simulink model "Ford_T3T6_ArchCnctnDigrm"  (R2016b)
settings: Solver=FixedStepDiscrete  StartTime=0.0  StopTime=10.0  RelTol=1e-3  EnableMultiTasking=on
libraries: canmsglib x15
(part 7 of 15)

== system Ford_T3T6_ArchCnctnDigrm/Vector Components Base Software/SYS ==
  AR001ABswM_BswM : Subsystem  Tag=0.0.X  Description=The BSW Mode Manager is the module that implements the part of the Vehicle Mode Management and Application Mode Management concept that resides in the BSW. Its responsibility is to arbitrate mode requests from application layer SW-Cs or other BSW modules based on simple rules, and perform actions based on the arbitration result.
      settings: AttributesFormatString=Version: %<Tag>
  AR001AComM_ComM : Subsystem  Tag=0.0.X  Description=The Communication Manager Module (COM Manager, ComM) is a component of the Basic Software (BSW). It is a Resource Manager, which encapsulates the control of the underlying communication services. The ComM module controls basic software modules relating to communication and not software components or runnable entities. The ComM module collects the bus communication access requests from communication requestors and coordinates the bus communication access requests. The purpose of the ComM module is: 1. Simplifying the usage of the bus communication stack for the user. This includes a simplified network management handling. 2. Coordinating the availability of the bus communication stack (allow sending and receiving of signals) of multiple independent software components on one ECU. 3. Offer an API to disable sending of signals to prevent the ECU from (actively) waking up the communication bus. 4. Controlling of more than one communication bus channel of an ECU by implementing a channel state machine for every channel. 5. Offering the possibility to force an ECU that keeps the bus awake to the ï¿½No Communicationï¿½ mode. 6. Simplifying the resource management by allocating all resources necessary for the requested Communication Mode.
      settings: AttributesFormatString=Version: %<Tag>
  AR001ADet_Det : Subsystem  Tag=0.0.X  Description=All detected development errors in the Basic Software are reported to this module. The API parameters allow for tracing source and kind of error: Module in which error has been detected, Function in which error has been detected, Type of error
      settings: AttributesFormatString=Version: %<Tag>
  AR001AWdgIf_WdgIf : Subsystem  Tag=0.0.X  Description=In case of more than one watchdog device and watchdog driver (e.g. both an internal software watchdog and an external hardware watchdog) being used on an ECU, this module allows the watchdog manager (or any other client of the watchdog) to select the correct watchdog driver - and thus the watchdog device - while retaining the API and functionality of the underlying driver.
      settings: AttributesFormatString=Version: %<Tag>
  AR001AWdgM_WdgM : Subsystem  Tag=0.0.X  Description=The Watchdog Manager is able to supervise the program execution abstracting from the triggering of hardware watchdog entities. The Watchdog Manager supervises the execution of a configurable number of socalled Supervised Entities. When it detects a violation of the configured temporal and/or logical constraints on program execution, it takes a number of configurable actions to recover from this failure. The watchdog Manager provides three mechanisms: 1. Alive supervision ï¿½ for supervision of timing of periodic software. 2. Deadline monitoring ï¿½ for aperiodic software. 3. Logical monitoring ï¿½ for supervision of the correctness of the execution sequence.
      settings: AttributesFormatString=Version: %<Tag>
  tag scope: BswM_RequestMode=global, ComM_RequestComMode=global, PortDefinedArgument_CheckpointReached=global, WdgM_ActivateSupervisionEntity=global, WdgM_CheckpointReached=global, WdgM_DeactivateSupervisionEntity=global
  wires:
  AR001ABswM_BswM/1(BswM_RequestMode) -> [BswM_RequestMode]
  AR001AComM_ComM/1(ComM_RequestComMode) -> [ComM_RequestComMode]
  AR001AWdgM_WdgM/1(PortDefinedArgument_CheckpointReached) -> [PortDefinedArgument_CheckpointReached]
  AR001AWdgM_WdgM/2(WdgM_ActivateSupervisionEntity) -> [WdgM_ActivateSupervisionEntity]
  AR001AWdgM_WdgM/3(WdgM_CheckpointReached) -> [WdgM_CheckpointReached]
  AR001AWdgM_WdgM/4(WdgM_DeactivateSupervisionEntity) -> [WdgM_DeactivateSupervisionEntity]

== system Ford_T3T6_ArchCnctnDigrm/Vehicle Com/CF049A_FordVehSpdArbn ==
  FordAbsModlPrsnt : Inport
  FordEscModlPrsnt : Inport  Port=2
  FordVehFrntLeWhlSpd : Inport  Port=3
  FordVehFrntLeWhlSpdVld : Inport  Port=4
  FordVehFrntRiWhlSpd : Inport  Port=5
  FordVehFrntRiWhlSpdVld : Inport  Port=6
  FordVehReLeWhlSpd : Inport  Port=7
  FordVehReLeWhlSpdVld : Inport  Port=8
  FordVehReRiWhlSpd : Inport  Port=9
  FordVehReRiWhlSpdVld : Inport  Port=10
  FordVehSpdBrkModl : Inport  Port=11
  FordVehSpdBrkModlLoQlyVld : Inport  Port=12
  FordVehSpdBrkModlVld : Inport  Port=13
  FordVehSpdEngModl : Inport  Port=14
  FordVehSpdEngModlLoQlyVld : Inport  Port=15
  FordVehSpdEngModlVld : Inport  Port=16
  FordVehTireCircum_GetErrorStatus : Inport  Port=17
  FordVehSpd : Outport
  FordVehSpdLoQly : Outport  Port=2
  FordVehSpdLoQlyVld : Outport  Port=3
  FordVehSpdVld : Outport  Port=4

== system Ford_T3T6_ArchCnctnDigrm/Vehicle Com/CF100A_FordCanSigVldFlgGenr ==
  ActvFrntSteerModlSteerWhlAgVldInt : Inport
  FordVehActvFrntSteerModSteerWhlAgRaw : Inport  Port=2
  FordVehGearLvrPosnRaw : Inport  Port=3
  FordVehGearPosnRaw : Inport  Port=4
  FordVehParkAidModlReqdAgRaw : Inport  Port=5
  FordVehParkAidModlReqdStsRaw : Inport  Port=6
  FordVehTrlrAgOffsDirRaw : Inport  Port=7
  FordVehTrlrAidIdnNrRaw : Inport  Port=8
  FordVehTrlrAidSetUpRaw : Inport  Port=9
  FordVehTrlrAidTrlrRvsGuidcStsRaw : Inport  Port=10
  FordVehTrlrEnaReqRaw : Inport  Port=11
  FordVehTrlrIdnTypRaw : Inport  Port=12
  FordVehTrlrRvsCnclReqRaw : Inport  Port=13
  FordVehTrlrRvsEnaRaw : Inport  Port=14
  FordVehTrlrRvsMsgTxtReqRaw : Inport  Port=15
  FordVehTrsmDesGearRaw : Inport  Port=16
  GearLvrPosnVldInt : Inport  Port=17
  GearPosnRawVldInt : Inport  Port=18
  ImgProcgDataPrsntInt : Inport  Port=19
  ParkAidModlReqdAgVldInt : Inport  Port=20
  ParkAidModlReqdStsVldInt : Inport  Port=21
  TrlrAidDataPrsntInt : Inport  Port=22
  TrlrAidDataThreePrsntInt : Inport  Port=23
  TrlrAidStsThreePrsntInt : Inport  Port=24
  TrsmDesGearRawVldInt : Inport  Port=25
  FordVehActvFrntSteerModSteerWhlAg : Outport
  FordVehActvParkAssiVld : Outport  Port=2
  FordVehGearLvrPosn : Outport  Port=3
  FordVehGearLvrPosnVld : Outport  Port=4
  FordVehGearPosn : Outport  Port=5
  FordVehParkAidModlReqdAg : Outport  Port=6
  FordVehParkAidModlReqdSts : Outport  Port=7
  FordVehTrlrAgOffsDir : Outport  Port=8
  FordVehTrlrAidIdnNr : Outport  Port=9
  FordVehTrlrAidSetUp : Outport  Port=10
  FordVehTrlrAidTrlrRvsGuidcSts : Outport  Port=11
  FordVehTrlrBackUpAssiEnaVld : Outport  Port=12
  FordVehTrlrBackUpAssiRvsVld : Outport  Port=13
  FordVehTrlrEnaReq : Outport  Port=14
  FordVehTrlrIdnTyp : Outport  Port=15
  FordVehTrlrRvsCnclReq : Outport  Port=16
  FordVehTrlrRvsEna : Outport  Port=17
  FordVehTrlrRvsMsgTxtReq : Outport  Port=18
  FordVehTrsmDesGear : Outport  Port=19

== system Ford_T3T6_ArchCnctnDigrm/Vehicle Com/Rx Messages ==
  Acc Pedal Posn : Subsystem
  Ambient Temperature : Subsystem
  Brake Data : Subsystem
  Evasive Steer Assist : Subsystem
  Lane Keep Asssist : Subsystem
  Lat and Long Acceleration : Subsystem
  Park Assist : Subsystem
  Pinion Data : Subsystem
  Steering Request Command : Subsystem
  Trailer Aid : Subsystem
  Transmission Data : Subsystem
  Vehicle Data : Subsystem
  Wheel Data : Subsystem
  Yaw Rate : Subsystem

== system Ford_T3T6_ArchCnctnDigrm/Vehicle Com/SF033A_VehSigCdng ==
  HwTq : Inport
  VehLatASerlCom : Inport  Port=2
  VehLatAVldSerlCom : Inport  Port=3
  VehLgtASerlCom : Inport  Port=4
  VehLgtAVldSerlCom : Inport  Port=5
  VehSpdOvrd : Inport  Port=6
  VehSpdOvrdEna : Inport  Port=7
  VehSpdSerlCom : Inport  Port=8
  VehSpdVldSerlCom : Inport  Port=9
  VehYawRateSerlCom : Inport  Port=10
  VehYawRateVldSerlCom : Inport  Port=11
  FltInj_f32 : Inport  Port=12
  VehLatA : Outport
  VehLatAEstimd : Outport  Port=2
  VehLatAEstimdVld : Outport  Port=3
  VehLatAVld : Outport  Port=4
  VehLgtA : Outport  Port=5
  VehLgtAVld : Outport  Port=6
  VehSpd : Outport  Port=7
  VehSpdVld : Outport  Port=8
  VehYawRate : Outport  Port=9
  VehYawRateVld : Outport  Port=10

== system Ford_T3T6_ArchCnctnDigrm/Vehicle Com/Tx Messages ==
  note: StePw_B_Rq
  note: VehVtrlrAid_B_Rq
  note: TrlrHitchLamp_D_Rqst
  note: SteMdule_D_Stat
  note: EPAS_Failure
  note: SteMdule_U_Meas
  note: SteMdule_I_Est
  note: DrvSte_Tq_Actl
  note: SteeringColumnTorque
  note: Veh_V_RqMxTrlrAid
  note: DrvSteActV_B_Stat
  note: Future MMs will be:
      | Msg 60E
      | 60F
      | 63A
      | 63B
      | 63D
      | 63E
      | 63F
      | 738
  note: To COM
  note: To COM
  note: To COM
  note: To COM
  note: To COM
  CAN Pack : canmsglib/CAN Pack  CANdbFile=C:\Users\nz3503\Desktop\Ford Architecture\FD1_CAN_P702_GASDHEV_MY21_V04.dbc  MsgList=SteeringPinion_Data_FD1  MsgName=SteeringPinion_Data_FD1  MsgIDType=Standard (11-bit identifier)  MsgIdentifier=126  MsgLength=8  SignalInfo=StePinAn_No_Cnt$44$4$2$2$1$0$1$0$0$15$#StePinAn_No_Cs$32$8$2$2$1$0$1$0$0$255$#StePinCompAnEst_D_Qf$42$2$2$2$1$0$1$0$0$3$#StePinComp_An_Est$24$15$2$2$1$0$1.000000e-01$-1600$-1600$1.676700e+03$#StePinRelInit_An_Sns$8$16$2$2$1$0$1.000000e-01$-3200$-3200$3.353300e+03$#StePw_B_Rq$23$1$2$2$1$0$1$0$0$1$#  NSignals=6  StartBits=str2num('[int32(44);int32(32);int32(42);int32(24);int32(8);int32(23)]')  SignalSizes=str2num('[int32(4);int32(8);int32(2);int32(15);int32(16);int32(1)]')  ByteOrders=str2num('[int32(2);int32(2);int32(2);int32(2);int32(2);int32(2)]')  DataTypes=str2num('[int32(2);int32(2);int32(2);int32(2);int32(2);int32(2)]')  MultiplexTypes=str2num('[int32(1);int32(1);int32(1);int32(1);int32(1);int32(1)]')  MultiplexValues=str2num('[double(0);double(0);double(0);double(0);double(0);double(0)]')  Factors=str2num('[double(1);double(1);double(1);double(1.000000e-01);double(1.000000e-01);double(1)]')  Offsets=str2num('[double(0);double(0);double(0);double(-1600);double(-3200);double(0)]')  Minimums=str2num('[double(0);double(0);double(0);double(-1600);double(-3200);double(0)]')  Maximums=str2num('[double(15);double(255);double(3);double(1.676700e+03);double(3.353300e+03);double(1)]')  Remote=off
      settings: DataFormat=CANdb specified signals
  CAN Pack1 : canmsglib/CAN Pack  CANdbFile=C:\Users\nz3503\Desktop\Ford Architecture\FD1_CAN_P702_GASDHEV_MY21_V04.dbc  MsgList=EPAS_INFO_FD1  MsgName=EPAS_INFO_FD1  MsgIDType=Standard (11-bit identifier)  MsgIdentifier=130  MsgLength=8  SignalInfo=DrvSteActv_B_Stat$10$1$2$2$1$0$1$0$0$1$#DrvSte_Tq_Actl$40$8$2$2$1$0$6.250000e-02$-8$-8$7.812500e+00$#EPAS_Failure$8$2$2$2$1$0$1$0$0$3$#SAPPAngleControlStat1$22$2$2$2$1$0$1$0$0$3$#SAPPAngleControlStat2$11$1$2$2$1$0$1$0$0$1$#SAPPAngleControlStat3$12$1$2$2$1$0$1$0$0$1$#SAPPAngleControlStat4$13$1$2$2$1$0$1$0$0$1$#SAPPAngleControlStat5$14$1$2$2$1$0$1$0$0$1$#SAPPAngleControlStat6$15$1$2$2$1$0$1$0$0$1$#SteMdule_D_Stat$53$3$2$2$1$0$1$0$0$7$#SteMdule_I_Est$26$12$2$2$1$0$5.000000e-02$-64$-64$1.407000e+02$#SteMdule_U_Meas$32$8$2$2$1$0$5.000000e-02$6$6$1.870000e+01$#SteeringColumnTorque$0$8$2$2$1$0$6.250000e-02$-8$-8$7.812500e+00$#TrlrHitchLamp_D_Rqst$24$1$2$2$1$0$1$0$0$1$#VehVTrlrAid_B_Rq$25$1$2$2$1$0$1$0$0$1$#Veh_V_RqMxTrlrAid$56$8$2$2$1$0$1.000000e-01$0$0$2.550000e+01$#  NSignals=16  StartBits=str2num('[int32(10);int32(40);int32(8);int32(22);int32(11);int32(12);int32(13);int32(14);int32(15);int32(53);int32(26);int32(32);int32(0);int32(24);int32(25);int32(56)]')  SignalSizes=str2num('[int32(1);int32(8);int32(2);int32(2);int32(1);int32(1);int32(1);int32(1);int32(1);int32(3);int32(12);int32(8);int32(8);int32(1);int32(1);int32(8)]')  ByteOrders=str2num('[int32(2);int32(2);int32(2);int32(2);int32(2);int32(2);int32(2);int32(2);int32(2);int32(2);int32(2);int32(2);int32(2);int32(2);int32(2);int32(2)]')  DataTypes=str2num('[int32(2);int32(2);int32(2);int32(2);int32(2);int32(2);int32(2);int32(2);int32(2);int32(2);int32(2);int32(2);int32(2);int32(2);int32(2);int32(2)]')  MultiplexTypes=str2num('[int32(1);int32(1);int32(1);int32(1);int32(1);int32(1);int32(1);int32(1);int32(1);int32(1);int32(1);int32(1);int32(1);int32(1);int32(1);int32(1)]')  MultiplexValues=str2num('[double(0);double(0);double(0);double(0);double(0);double(0);double(0);double(0);double(0);double(0);double(0);double(0);double(0);double(0);double(0);double(0)]')  Factors=str2num('[double(1);double(6.250000e-02);double(1);double(1);double(1);double(1);double(1);double(1);double(1);double(1);double(5.000000e-02);double(5.000000e-02);double(6.250000e-02);double(1);double(1);double(1.000000e-01)]')  Offsets=str2num('[double(0);double(-8);double(0);double(0);double(0);double(0);double(0);double(0);double(0);double(0);double(-64);double(6);double(-8);double(0);double(0);double(0)]')  Minimums=str2num('[double(0);double(-8);double(0);double(0);double(0);double(0);double(0);double(0);double(0);double(0);double(-64);double(6);double(-8);double(0);double(0);double(0)]')  Maximums=str2num('[double(1);double(7.812500e+00);double(3);double(3);double(1);double(1);double(1);double(1);double(1);double(7);double(1.407000e+02);double(1.870000e+01);double(7.812500e+00);double(1);double(1);double(2.550000e+01)]')  Remote=off
      settings: DataFormat=CANdb specified signals
  CAN Pack2 : canmsglib/CAN Pack  CANdbFile=C:\Users\nz3503\Desktop\Ford Architecture\FD1_CAN_P702_GASDHEV_MY21_V04.dbc  MsgList=TrailerAid_Data2_FD1  MsgName=TrailerAid_Data2_FD1  MsgIDType=Standard (11-bit identifier)  MsgIdentifier=1047  MsgLength=8  SignalInfo=EsaOn_B_Stat$23$1$2$2$1$0$1$0$0$1$#HitchToTrlrAxle_L_Calc$15$9$2$2$1$0$2.540000e-02$0$0$1.297940e+01$#LatCtlLim_D_Stat$21$2$2$2$1$0$1$0$0$3$#LatCtlSte_D_Stat$18$3$2$2$1$0$1$0$0$7$#SelDrvMdeSte_D_Stat$16$2$2$2$1$0$1$0$0$3$#TrlrAidEnbl_D2_Stat$29$3$2$2$1$0$1$0$0$7$#TrlrAidMsgTxt_D2_Rq$9$6$2$2$1$0$1$0$0$63$#TrlrAidSetup_D2_Stat$45$3$2$2$1$0$1$0$0$7$#TrlrAidTrgtId_No_Rq$40$5$2$2$1$0$1$0$0$31$#TrlrAidTrlrId_No_Rq$60$4$2$2$1$0$1$0$0$15$#TrlrAnOffst_An2_Calc$32$8$2$2$1$0$5.000000e-01$-64$-64$6.350000e+01$#TrlrAn_An_MxCalc$49$7$2$2$1$0$1$0$0$127$#TrlrAn_An_WarnCalc$24$5$2$2$1$0$1$0$0$31$#  NSignals=13  StartBits=str2num('[int32(23);int32(15);int32(21);int32(18);int32(16);int32(29);int32(9);int32(45);int32(40);int32(60);int32(32);int32(49);int32(24)]')  SignalSizes=str2num('[int32(1);int32(9);int32(2);int32(3);int32(2);int32(3);int32(6);int32(3);int32(5);int32(4);int32(8);int32(7);int32(5)]')  ByteOrders=str2num('[int32(2);int32(2);int32(2);int32(2);int32(2);int32(2);int32(2);int32(2);int32(2);int32(2);int32(2);int32(2);int32(2)]')  DataTypes=str2num('[int32(2);int32(2);int32(2);int32(2);int32(2);int32(2);int32(2);int32(2);int32(2);int32(2);int32(2);int32(2);int32(2)]')  MultiplexTypes=str2num('[int32(1);int32(1);int32(1);int32(1);int32(1);int32(1);int32(1);int32(1);int32(1);int32(1);int32(1);int32(1);int32(1)]')  MultiplexValues=str2num('[double(0);double(0);double(0);double(0);double(0);double(0);double(0);double(0);double(0);double(0);double(0);double(0);double(0)]')  Factors=str2num('[double(1);double(2.540000e-02);double(1);double(1);double(1);double(1);double(1);double(1);double(1);double(1);double(5.000000e-01);double(1);double(1)]')  Offsets=str2num('[double(0);double(0);double(0);double(0);double(0);double(0);double(0);double(0);double(0);double(0);double(-64);double(0);double(0)]')  Minimums=str2num('[double(0);double(0);double(0);double(0);double(0);double(0);double(0);double(0);double(0);double(0);double(-64);double(0);double(0)]')  Maximums=str2num('[double(1);double(1.297940e+01);double(3);double(7);double(3);double(7);double(63);double(7);double(31);double(15);double(6.350000e+01);double(127);double(31)]')  Remote=off
      settings: DataFormat=CANdb specified signals
  CAN Pack3 : canmsglib/CAN Pack  CANdbFile=C:\Users\nz3503\Desktop\Ford Architecture\FD1_CAN_P702_GASDHEV_MY21_V04.dbc  MsgList=PCM_AutoSar_NetworkMgt_FD1  MsgName=PCM_AutoSar_NetworkMgt_FD1  MsgIDType=Standard (11-bit identifier)  MsgIdentifier=1429  MsgLength=8  SignalInfo=PCM_AutoSarNMControl$8$8$2$2$1$0$1$0$0$255$#PCM_AutoSarNMNodeId$0$8$2$2$1$0$1$0$0$255$#PCM_AutoSarNMReserved1$16$8$2$2$1$0$1$0$0$255$#PCM_AutoSarNMReserved2$24$8$2$2$1$0$1$0$0$255$#PCM_AutoSarNMReserved3$48$8$2$2$1$0$1$0$0$255$#PCM_AutoSarNMReserved4$56$8$2$2$1$0$1$0$0$255$#PCM_GWNMProxy$40$8$2$2$1$0$1$0$0$255$#PCM_GWOnBoardTester$32$8$2$2$1$0$1$0$0$255$#  NSignals=8  StartBits=str2num('[int32(8);int32(0);int32(16);int32(24);int32(48);int32(56);int32(40);int32(32)]')  SignalSizes=str2num('[int32(8);int32(8);int32(8);int32(8);int32(8);int32(8);int32(8);int32(8)]')  ByteOrders=str2num('[int32(2);int32(2);int32(2);int32(2);int32(2);int32(2);int32(2);int32(2)]')  DataTypes=str2num('[int32(2);int32(2);int32(2);int32(2);int32(2);int32(2);int32(2);int32(2)]')  MultiplexTypes=str2num('[int32(1);int32(1);int32(1);int32(1);int32(1);int32(1);int32(1);int32(1)]')  MultiplexValues=str2num('[double(0);double(0);double(0);double(0);double(0);double(0);double(0);double(0)]')  Factors=str2num('[double(1);double(1);double(1);double(1);double(1);double(1);double(1);double(1)]')  Offsets=str2num('[double(0);double(0);double(0);double(0);double(0);double(0);double(0);double(0)]')  Minimums=str2num('[double(0);double(0);double(0);double(0);double(0);double(0);double(0);double(0)]')  Maximums=str2num('[double(255);double(255);double(255);double(255);double(255);double(255);double(255);double(255)]')  Remote=off
      settings: DataFormat=CANdb specified signals
  CAN Pack4 : canmsglib/CAN Pack  CANdbFile=C:\Users\nz3503\Desktop\Ford Architecture\FD1_CAN_P702_GASDHEV_MY21_V04.dbc  MsgList=Lane_Assist_Data3_FD1  MsgName=Lane_Assist_Data3_FD1  MsgIDType=Standard (11-bit identifier)  MsgIdentifier=972  MsgLength=8  SignalInfo=LaActAvail_D_Actl$4$2$2$2$1$0$1$0$0$3$#LaActDeny_B_Actl$6$1$2$2$1$0$1$0$0$1$#LaHandsOff_B_Actl$7$1$2$2$1$0$1$0$0$1$#LsmcBrkDecelEnbl_D_Rq$0$2$2$2$1$0$1$0$0$3$#LsmcBrk_Tq_Rq$19$13$2$2$1$0$4$0$0$32764$#TjaHandsOnCnfdnc_B_Est$3$1$2$2$1$0$1$0$0$1$#TrlrAn_An_TrgtCalc$24$8$2$2$1$0$1$-128$-128$127$#  NSignals=7  StartBits=str2num('[int32(4);int32(6);int32(7);int32(0);int32(19);int32(3);int32(24)]')  SignalSizes=str2num('[int32(2);int32(1);int32(1);int32(2);int32(13);int32(1);int32(8)]')  ByteOrders=str2num('[int32(2);int32(2);int32(2);int32(2);int32(2);int32(2);int32(2)]')  DataTypes=str2num('[int32(2);int32(2);int32(2);int32(2);int32(2);int32(2);int32(2)]')  MultiplexTypes=str2num('[int32(1);int32(1);int32(1);int32(1);int32(1);int32(1);int32(1)]')  MultiplexValues=str2num('[double(0);double(0);double(0);double(0);double(0);double(0);double(0)]')  Factors=str2num('[double(1);double(1);double(1);double(1);double(4);double(1);double(1)]')  Offsets=str2num('[double(0);double(0);double(0);double(0);double(0);double(0);double(-128)]')  Minimums=str2num('[double(0);double(0);double(0);double(0);double(0);double(0);double(-128)]')  Maximums=str2num('[double(3);double(1);double(1);double(3);double(32764);double(1);double(127)]')  Remote=off
      settings: DataFormat=CANdb specified signals
  MM518A_FordMsg417BusHiSpd : Subsystem  Tag=4.0.X  Description=The purpose of the Ford Message 417 Bus High Speed function is to transmit Electric Power Assisted Steering information to other vehicle modules.
      settings: AttributesFormatString=Version: %<Tag>
  MM519A_FordMsg5B5BusHiSpd : Subsystem  Tag=2.0.0  Description=The purpose of the Ford Message 5B5 Bus High Speed function is to transmit Electric Power Assisted Steering information to other vehicle modules.
      settings: AttributesFormatString=Version: %<Tag>
  MM531A_FordMsg07EBusHiSpd : Subsystem  Tag=2.0.0  Description=Ford Message 07E Bus High Speed provides other vehicle modules with Steering Pinion Angle signals
      settings: AttributesFormatString=Version: %<Tag>
  MM532A_FordMsg082BusHiSpd : Subsystem  Tag=2.0.0  Description=The purpose of the Ford Message 082 Bus High Speed function is to transmitElectric Power Assisted Steering information to other vehicle modules.
      settings: AttributesFormatString=Version: %<Tag>
  MM533A_FordMsg3CCBusHiSpd : Subsystem  Tag=4.0.X  Description=The purpose of the Ford Message 3CC Bus High Speed function is to transmit Electric Power Assisted Steering information to other vehicle modules.
      settings: AttributesFormatString=Version: %<Tag>
  Terminator{,1..49} (50 alike) : Terminator
  wires:
  MM519A_FordMsg5B5BusHiSpd/1(PSCM_AutoSarNMControl) -> Terminator6/1
  MM519A_FordMsg5B5BusHiSpd/2(PSCM_AutoSarNMNodeId) -> Terminator7/1
  MM519A_FordMsg5B5BusHiSpd/3(PSCM_AutoSarNMReserved1) -> Terminator8/1
  MM519A_FordMsg5B5BusHiSpd/4(PSCM_AutoSarNMReserved2) -> Terminator9/1
  MM519A_FordMsg5B5BusHiSpd/5(PSCM_AutoSarNMReserved3) -> Terminator10/1
  MM519A_FordMsg5B5BusHiSpd/6(PSCM_AutoSarNMReserved4) -> Terminator11/1
  MM519A_FordMsg5B5BusHiSpd/7(PSCM_GWNMProxy) -> Terminator12/1
  MM519A_FordMsg5B5BusHiSpd/8(PSCM_GWOnBoardTester) -> Terminator13/1
  [FordCmpdHwPosn] -> MM531A_FordMsg07EBusHiSpd/1(CmpdSteerPinionAg)
  [FordCmpdHwPosnQlyFac] -> MM531A_FordMsg07EBusHiSpd/2(CmpdSteerPinionAgQlyFac)
  [FordVehSteerPwrReq] -> MM531A_FordMsg07EBusHiSpd/3(FordVehSteerPwrReq)
  [FordRelHwPosn] -> MM531A_FordMsg07EBusHiSpd/4(RelSteerPinionAg)
  MM531A_FordMsg07EBusHiSpd/1(Ford_StePinAn_No_Cnt) -> Terminator14/1
  MM531A_FordMsg07EBusHiSpd/2(Ford_StePinAn_No_Cs) -> Terminator15/1
  MM531A_FordMsg07EBusHiSpd/3(Ford_StePinCompAnEst_D_Qf1) -> Terminator16/1
  MM531A_FordMsg07EBusHiSpd/4(Ford_StePinComp_An_Est) -> Terminator17/1
  MM531A_FordMsg07EBusHiSpd/5(Ford_StePinRelInit_An_Sns) -> Terminator18/1
  MM531A_FordMsg07EBusHiSpd/6(Ford_StePw_B_Rq1) -> Terminator19/1
  [FordEpsCurr] -> MM532A_FordMsg082BusHiSpd/1(ElecPwrSteerCurr)
  [FordEpsVltg] -> MM532A_FordMsg082BusHiSpd/2(ElecPwrSteerVltg)
  [FordEpsFailr] -> MM532A_FordMsg082BusHiSpd/3(FordElecPwrAssidSteerFailr)
  [FordSteerModlSts] -> MM532A_FordMsg082BusHiSpd/4(FordSteerModlSts)
  [FordVehDrvrSteerActvnSts] -> MM532A_FordMsg082BusHiSpd/5(FordVehDrvrSteerActvnSts)
  [FordVehDrvrSteerTqReq] -> MM532A_FordMsg082BusHiSpd/6(FordVehDrvrSteerTqReq)
  [FordVehReCamrLiSts] -> MM532A_FordMsg082BusHiSpd/7(FordVehReCamrLiSts)
  [SemiAutParlParkAgCtrlSts1] -> MM532A_FordMsg082BusHiSpd/8(FordVehSAPPAgCtrlSts1)
  [SemiAutParlParkAgCtrlSts2] -> MM532A_FordMsg082BusHiSpd/9(FordVehSAPPAgCtrlSts2)
  [SemiAutParlParkAgCtrlSts3] -> MM532A_FordMsg082BusHiSpd/10(FordVehSAPPAgCtrlSts3)
  [SemiAutParlParkAgCtrlSts4] -> MM532A_FordMsg082BusHiSpd/11(FordVehSAPPAgCtrlSts4)
  [SemiAutParlParkAgCtrlSts5] -> MM532A_FordMsg082BusHiSpd/12(FordVehSAPPAgCtrlSts5)
  [SemiAutParlParkAgCtrlSts6] -> MM532A_FordMsg082BusHiSpd/13(FordVehSAPPAgCtrlSts6)
  [FordVehVelMaxReqTrlrAid] -> MM532A_FordMsg082BusHiSpd/14(FordVehVelMaxReqTrlrAid)
  [FordVehVelTrlrAidReq] -> MM532A_FordMsg082BusHiSpd/15(FordVehVelTrlrAidReq)
  [FordInpTqRaw] -> MM532A_FordMsg082BusHiSpd/16(InpTqRaw)
  MM532A_FordMsg082BusHiSpd/1(Ford_DrvSteActv_B_Stat1) -> Terminator24/1
  MM532A_FordMsg082BusHiSpd/2(Ford_DrvSte_Tq_Actl) -> Terminator25/1
  MM532A_FordMsg082BusHiSpd/3(Ford_EPAS_Failure1) -> Terminator26/1
  MM532A_FordMsg082BusHiSpd/4(Ford_SAPPAngleControlStat1_1) -> Terminator27/1
  MM532A_FordMsg082BusHiSpd/5(Ford_SAPPAngleControlStat2_1) -> Terminator20/1
  MM532A_FordMsg082BusHiSpd/6(Ford_SAPPAngleControlStat3_1) -> Terminator21/1
  MM532A_FordMsg082BusHiSpd/7(Ford_SAPPAngleControlStat4_1) -> Terminator22/1
  MM532A_FordMsg082BusHiSpd/8(Ford_SAPPAngleControlStat5_1) -> Terminator23/1
  MM532A_FordMsg082BusHiSpd/9(Ford_SAPPAngleControlStat6_1) -> Terminator32/1
  MM532A_FordMsg082BusHiSpd/10(Ford_SteMdule_D_Stat1) -> Terminator33/1
  MM532A_FordMsg082BusHiSpd/11(Ford_SteMdule_I_Est) -> Terminator28/1
  MM532A_FordMsg082BusHiSpd/12(Ford_SteMdule_U_Meas) -> Terminator29/1
  MM532A_FordMsg082BusHiSpd/13(Ford_SteeringColumnTorque) -> Terminator30/1
  MM532A_FordMsg082BusHiSpd/14(Ford_TrlrHitchLamp_D_Rqst1) -> Terminator31/1
  MM532A_FordMsg082BusHiSpd/15(Ford_VehVTrlrAid_B_Rq1) -> Terminator34/1
  MM532A_FordMsg082BusHiSpd/16(Ford_Veh_V_RqMxTrlrAid) -> Terminator35/1
  [FordVehEvasSteerAssiSts] -> MM518A_FordMsg417BusHiSpd/1(FordVehEvasSteerAssiSts)
  [FordVehLatCtrlLimSts] -> MM518A_FordMsg417BusHiSpd/2(FordVehLatCtrlLimSts)
  [FordVehLatCtrlSteerSts] -> MM518A_FordMsg417BusHiSpd/3(FordVehLatCtrlSteerSts)
  [FordVehSelDrvModSteerSts] -> MM518A_FordMsg417BusHiSpd/4(FordVehSelDrvModSteerSts)
  [FordVehTrlrAgMax] -> MM518A_FordMsg417BusHiSpd/5(FordVehTrlrAidAgMax)
  [FordVehTrlrAgOffs] -> MM518A_FordMsg417BusHiSpd/6(FordVehTrlrAidAgOffs)
  [FordVehTrlrAidAgWarn] -> MM518A_FordMsg417BusHiSpd/7(FordVehTrlrAidAgWarn)
  [FordVehTrlrAidEnaSts] -> MM518A_FordMsg417BusHiSpd/8(FordVehTrlrAidEnaSts)
  [FordVehHitchToTrlrAxle] -> MM518A_FordMsg417BusHiSpd/9(FordVehTrlrAidHitchToAxle)
  [FordVehTrlrAidMsgTxtReq] -> MM518A_FordMsg417BusHiSpd/10(FordVehTrlrAidMsgTxtReq)
  [FordVehTrlrAidSetUpSts] -> MM518A_FordMsg417BusHiSpd/11(FordVehTrlrAidSetUp)
  [FordVehTrlrAidTarIdnReq] -> MM518A_FordMsg417BusHiSpd/12(FordVehTrlrAidTarIdn)
  [FordVehTrlrAidTrlredReq] -> MM518A_FordMsg417BusHiSpd/13(FordVehTrlrAidTrlrIdn)
  MM518A_FordMsg417BusHiSpd/1(Ford_EsaOn_B_Stat1) -> Terminator/1
  MM518A_FordMsg417BusHiSpd/2(Ford_HitchToTrlrAxle_L_Calc) -> Terminator1/1
  MM518A_FordMsg417BusHiSpd/3(Ford_LatCtlLim_D_Stat1) -> Terminator2/1
  MM518A_FordMsg417BusHiSpd/4(Ford_LatCtlSte_D_Stat1) -> Terminator3/1
  MM518A_FordMsg417BusHiSpd/5(Ford_SelDrvMdeSte_D_Stat1) -> Terminator4/1
  MM518A_FordMsg417BusHiSpd/6(Ford_TrlrAidEnbl_D2_Stat1) -> Terminator5/1
  MM518A_FordMsg417BusHiSpd/7(Ford_TrlrAidMsgTxt_D2_Rq1) -> Terminator41/1
  MM518A_FordMsg417BusHiSpd/8(Ford_TrlrAidSetup_D2_Stat1) -> Terminator42/1
  MM518A_FordMsg417BusHiSpd/9(Ford_TrlrAidTrgtId_No_Rq) -> Terminator43/1
  MM518A_FordMsg417BusHiSpd/10(Ford_TrlrAidTrlrId_No_Rq) -> Terminator44/1
  MM518A_FordMsg417BusHiSpd/11(Ford_TrlrAnOffst_An2_Calc) -> Terminator45/1
  MM518A_FordMsg417BusHiSpd/12(Ford_TrlrAn_An_MxCalc) -> Terminator46/1
  MM518A_FordMsg417BusHiSpd/13(Ford_TrlrAn_An_WarnCalc) -> Terminator47/1
  [FordVehLaneAssiAvl] -> MM533A_FordMsg3CCBusHiSpd/1(FordVehLaneAssiAvl)
  [FordVehLaneAssiHandsOff] -> MM533A_FordMsg3CCBusHiSpd/2(FordVehLaneAssiHandsOff)
  [FordVehLaneAssiRejctn] -> MM533A_FordMsg3CCBusHiSpd/3(FordVehLaneAssiRejctn)
  [FordVehLoSpdMtnCtrlBrkDecelEnaReq] -> MM533A_FordMsg3CCBusHiSpd/4(FordVehLoSpdMtnCtrlBrkDecelEna)
  [FordVehLoSpdMtnCtrlBrkTqReq] -> MM533A_FordMsg3CCBusHiSpd/5(FordVehLoSpdMtnCtrlBrkTqReq)
  [FordVehTrfcJamAvdncHandsOnConf] -> MM533A_FordMsg3CCBusHiSpd/6(FordVehTrfcJamAvdHandsOnConf)
  [FordVehTrlrAgTarCalcn] -> MM533A_FordMsg3CCBusHiSpd/7(FordVehTrlrAgTarCalcn)
  MM533A_FordMsg3CCBusHiSpd/1(Ford_LaActAvail_D_Actl1) -> Terminator36/1
  MM533A_FordMsg3CCBusHiSpd/2(Ford_LaActDeny_B_Actl1) -> Terminator37/1
  MM533A_FordMsg3CCBusHiSpd/3(Ford_LaHandsOff_B_Actl1) -> Terminator38/1
  MM533A_FordMsg3CCBusHiSpd/4(Ford_LsmcBrkDecelEnbl_D_Rq1) -> Terminator39/1
  MM533A_FordMsg3CCBusHiSpd/5(Ford_LsmcBrk_Tq_Rq) -> Terminator40/1
  MM533A_FordMsg3CCBusHiSpd/7(Ford_TrlrAn_An_TrgtCalc) -> Terminator49/1
  MM533A_FordMsg3CCBusHiSpd/6(Ford_TjaHandsOnCnfdnc_B_Est1) -> Terminator48/1

== system Ford_T3T6_ArchCnctnDigrm/Calculate Motor Voltage Command/Motor Control/SF101A_MotQuadDetn ==
  MotAgCumvAlgndMrf : Inport
  MotTqCmd : Inport  Port=2
  MotDirInsts : Outport
  MotQuad : Outport  Port=2

== system Ford_T3T6_ArchCnctnDigrm/Calculate Motor Voltage Command/Motor Control/SF102A_MotCtrlPrmEstimn ==
  DualEcuFltMtgtnEna : Inport
  MotAndThermProtnLoaMod : Inport  Port=2
  MotCurrDaxCmd : Inport  Port=3
  MotCurrQaxCmd : Inport  Port=4
  MotFetT : Inport  Port=5
  MotMagT : Inport  Port=6
  MotWidgT : Inport  Port=7
  MotPrmNom_GetErrorStatus : Inport  Port=8
  MotPrmNom_SetRamBlockStatus : Inport  Port=9
  MotBackEmfConEstimd : Outport
  MotInduDaxEstimd : Outport  Port=2
  MotInduDaxEstimdIvs : Outport  Port=3
  MotInduQaxEstimd : Outport  Port=4
  MotInduQaxEstimdIvs : Outport  Port=5
  MotREstimd : Outport  Port=6
  GetMotPrmNomEol : Outport  Port=7
  SetMotPrmNomEol : Outport  Port=8

== system Ford_T3T6_ArchCnctnDigrm/Calculate Motor Voltage Command/Motor Control/SF103A_MotRefMdl ==
  BrdgVltg : Inport
  DualEcuMotCtrlMtgtnEna : Inport  Port=2
  MotAndThermProtnLoaMod : Inport  Port=3
  MotBackEmfConEstimd : Inport  Port=4
  MotInduDaxEstimd : Inport  Port=5
  MotInduQaxEstimd : Inport  Port=6
  MotQuad : Inport  Port=7
  MotREstimd : Inport  Port=8
  MotTqCmdMrfScad : Inport  Port=9
  MotVelMrf : Inport  Port=10
  MotBackEmfVltg : Outport
  MotCurrAg : Outport  Port=2
  MotCurrDaxCmd : Outport  Port=3
  MotCurrDaxMax : Outport  Port=4
  MotCurrQaxCmd : Outport  Port=5
  MotReacncDax : Outport  Port=6
  MotReacncQax : Outport  Port=7
  MotVltgDaxFf : Outport  Port=8
  MotVltgDaxFfStat : Outport  Port=9
  MotVltgQaxFf : Outport  Port=10
  MotVltgQaxFfStat : Outport  Port=11
  MotVltgSatnIndFf : Outport  Port=12

== system Ford_T3T6_ArchCnctnDigrm/Calculate Motor Voltage Command/Motor Control/SF104A_MotCurrRegCfg ==
  DualEcuMotCtrlMtgtnEna : Inport
  MotAndThermProtnLoaMod : Inport  Port=2
  MotCurrEolCalSt : Inport  Port=3
  MotInduDaxEstimd : Inport  Port=4
  MotInduQaxEstimd : Inport  Port=5
  MotREstimd : Inport  Port=6
  MotVelMrf : Inport  Port=7
  VehSpd : Inport  Port=8
  MotAgElecDly : Outport
  MotDampgDax : Outport  Port=2
  MotDampgQax : Outport  Port=3
  MotIntglGainDax : Outport  Port=4
  MotIntglGainQax : Outport  Port=5
  MotPropGainDax : Outport  Port=6
  MotPropGainQax : Outport  Port=7

== system Ford_T3T6_ArchCnctnDigrm/Calculate Motor Voltage Command/Motor Control/SF105A_MotCurrRegVltgLimr ==
  MotCtrlMotAndThermProtnLoaMod : Inport
  MotCtrlMotInduDaxEstimdIvs : Inport  Port=2
  MotCtrlMotInduQaxEstimdIvs : Inport  Port=3
  MotCtrlMotREstimd : Inport  Port=4
  MotCtrlBrdgVltg : Inport  Port=5
  MotCtrlDualEcuMotCtrlMtgtnEna : Inport  Port=6
  MotCtrlMotAgElecDly : Inport  Port=7
  MotCtrlMotBackEmfVltg : Inport  Port=8
  MotCtrlMotCurrDax : Inport  Port=9
  MotCtrlMotCurrDaxCmd : Inport  Port=10
  MotCtrlMotCurrDaxMax : Inport  Port=11
  MotCtrlMotCurrQax : Inport  Port=12
  MotCtrlMotCurrQaxCmd : Inport  Port=13
  MotCtrlMotCurrQaxCoggCmd : Inport  Port=14
  MotCtrlMotCurrQaxRplCmd : Inport  Port=15
  MotCtrlMotDampgDax : Inport  Port=16
  MotCtrlMotDampgQax : Inport  Port=17
  MotCtrlMotIntglGainDax : Inport  Port=18
  MotCtrlMotIntglGainQax : Inport  Port=19
  MotCtrlMotPropGainDax : Inport  Port=20
  MotCtrlMotPropGainQax : Inport  Port=21
  MotCtrlMotReacncDax : Inport  Port=22
  MotCtrlMotReacncQax : Inport  Port=23
  MotCtrlMotVltgDaxFf : Inport  Port=24
  MotCtrlMotVltgQaxFf : Inport  Port=25
  MotCtrlSysSt : Inport  Port=26
  MotCtrlMotCurrQaxCmdFinal : Outport
  MotCtrlMotModlnIdx : Outport  Port=2
  MotCtrlMotPhaAdv : Outport  Port=3
  MotCtrlMotVltgDax : Outport  Port=4
  MotCtrlMotVltgQax : Outport  Port=5

== system Ford_T3T6_ArchCnctnDigrm/Calculate Motor Voltage Command/Motor Control/SF106A_MotRplCoggCfg ==
  MotBackEmfConEstimd : Inport
  MotCurrDaxCmd : Inport  Port=2
  MotCurrQaxCmd : Inport  Port=3
  MotInduDaxEstimd : Inport  Port=4
  MotInduQaxEstimd : Inport  Port=5
  MotTqCmdMrfScad : Inport  Port=6
  MotVelMrf : Inport  Port=7
  MotVltgSatnIndFf : Inport  Port=8
  MotRplCoggPrm_GetErrorStatus : Inport  Port=9
  MotRplCoggPrm_SetRamBlockStatus : Inport  Port=10
  MotAgElecDlyRpl : Outport
  MotCurrQaxToMotTqGain : Outport  Port=2
  MotTqRplCoggOrder1Mgn : Outport  Port=3
  MotTqRplCoggOrder1Pha : Outport  Port=4
  MotTqRplCoggOrder2Mgn : Outport  Port=5
  MotTqRplCoggOrder2Pha : Outport  Port=6
  MotTqRplCoggOrder3Mgn : Outport  Port=7
  MotTqRplCoggOrder3Pha : Outport  Port=8
  GetMotRplCoggPrm : Outport  Port=9
  SetMotRplCoggPrm : Outport  Port=10

== system Ford_T3T6_ArchCnctnDigrm/Calculate Motor Voltage Command/Motor Control/SF107A_MotRplCoggCmd ==
  MotCtrlMotAgElec : Inport
  MotCtrlMotAgElecDlyRpl : Inport  Port=2
  MotCtrlMotCurrQaxToMotTqGain : Inport  Port=3
  MotCtrlMotElecMeclPolarity : Inport  Port=4
  MotCtrlMotTqRplCoggOrder1Mgn : Inport  Port=5
  MotCtrlMotTqRplCoggOrder1Pha : Inport  Port=6
  MotCtrlMotTqRplCoggOrder2Mgn : Inport  Port=7
  MotCtrlMotTqRplCoggOrder2Pha : Inport  Port=8
  MotCtrlMotTqRplCoggOrder3Mgn : Inport  Port=9
  MotCtrlMotTqRplCoggOrder3Pha : Inport  Port=10
  MotCoggCmdY_GetErrorStatus : Inport  Port=11
  MotCoggCmdY_SetRamBlockStatus : Inport  Port=12
  MotCtrlMotCurrQaxCoggCmd : Outport
  MotCtrlMotCurrQaxRplCmd : Outport  Port=2
  GetMotCoggCmdPrm : Outport  Port=3
  SetMotCoggCmdPrm : Outport  Port=4

== system Ford_T3T6_ArchCnctnDigrm/Complex Drivers/Platform Config/CM107B_GuardCfgAndDiagc ==

== system Ford_T3T6_ArchCnctnDigrm/Complex Drivers/Platform Config/CM201A_DmaCfgAndUse ==
  MotCtrlMgr_MotCtrlToTwoMilliSec_Rec : Inport
  MotCtrlMgr_TwoMilliSecToMotCtrl_Rec : Inport  Port=2
  Adc1CfgAndUseAdc1EnaCnvn : Inport  Port=3
  ClrErrInjReg : Inport  Port=4
  GetRefTmr1MicroSec32bit : Inport  Port=5
  GetTiSpan1MicroSec32bit : Inport  Port=6
  ReadErrInjReg : Inport  Port=7
  StrtErrInjCntr : Inport  Port=8
  MotCtrlAdc0RawRes : Outport
  MotCtrlAdc1RawRes : Outport  Port=2
  MotCtrlMgr_MotCtrlFromTwoMilliSec_Rec : Outport  Port=3
  MotCtrlMgr_TwoMilliSecFromMotCtrl_Rec : Outport  Port=4
  DmaEna2MilliSecToMotCtrlTrf : Outport  Port=5
  DmaWaitForMotCtrlTo2MilliSecTrf : Outport  Port=6
  InjDmaErr : Outport  Port=7
  InjMcuDiagcErr : Outport  Port=8

== system Ford_T3T6_ArchCnctnDigrm/Complex Drivers/Platform Config/CM301A_Adcf0CfgAndUse ==
  MotCtrlAdcDiagcEndPtrOutp : Inport
  MotCtrlAdcDiagcStrtPtrOutp : Inport  Port=2

== system Ford_T3T6_ArchCnctnDigrm/Complex Drivers/Platform Config/CM321A_Adcf1CfgAndUse ==
  AdcDiagcEndPtrOutp : Inport
  AdcDiagcStrtPtrOutp : Inport  Port=2
  Adcf1EnaCnvn : Outport

== system Ford_T3T6_ArchCnctnDigrm/Complex Drivers/Platform Config/ES102A_PolarityCfg ==
  PolarityCfgSaved_SetRamBlockStatus : Inport
  AssiMechPolarity : Outport
  HwAgAPolarity : Outport  Port=2
  HwAgBPolarity : Outport  Port=3
  HwAgCPolarity : Outport  Port=4
  HwAgDPolarity : Outport  Port=5
  HwAgEPolarity : Outport  Port=6
  HwAgFPolarity : Outport  Port=7
  HwAgGPolarity : Outport  Port=8
  HwAgHPolarity : Outport  Port=9
  HwTqAPolarity : Outport  Port=10
  HwTqBPolarity : Outport  Port=11
  HwTqCPolarity : Outport  Port=12
  HwTqDPolarity : Outport  Port=13
  HwTqEPolarity : Outport  Port=14
  HwTqFPolarity : Outport  Port=15
  HwTqGPolarity : Outport  Port=16
  HwTqHPolarity : Outport  Port=17
  MotAgMeclAPolarity : Outport  Port=18
  MotAgMeclBPolarity : Outport  Port=19
  MotAgMeclCPolarity : Outport  Port=20
  MotAgMeclDPolarity : Outport  Port=21
  MotAgMeclEPolarity : Outport  Port=22
  MotAgMeclFPolarity : Outport  Port=23
  MotAgMeclGPolarity : Outport  Port=24
  MotAgMeclHPolarity : Outport  Port=25
  MotElecMeclPolarity : Outport  Port=26
  PolarityCfgRead : Outport  Port=27
  PolarityCfgWr : Outport  Port=28

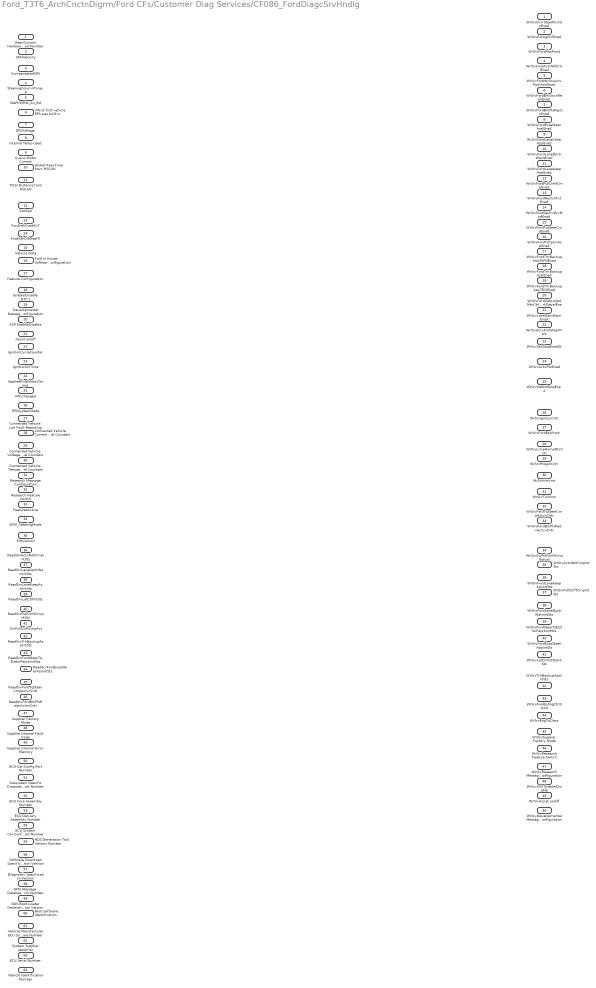
== system Ford_T3T6_ArchCnctnDigrm/Ford CFs/Customer Diag Services/CF086_FordDiagcSrvHndlg ==
  Gear/Column Hardware Part Number : Inport  OutMin=[0]  OutMax=[3]  OutDataTypeStr=uint8  Unit=Cnt
  SPAVelocity : Inport  Port=2  OutMin=[0]  OutMax=[3]  OutDataTypeStr=uint8  Unit=Cnt
  CompensatedSPA : Inport  Port=3  OutMin=[0]  OutMax=[3]  OutDataTypeStr=uint8  Unit=Cnt
  SteeringColumnTorque : Inport  Port=4  OutMin=[0]  OutMax=[3]  OutDataTypeStr=uint8  Unit=Cnt
  StePinOffst_An_Est : Inport  Port=5  OutMin=[0]  OutMax=[3]  OutDataTypeStr=uint8  Unit=Cnt
  VIN of first vehicle EPS was built in : Inport  Port=6  OutMin=[0]  OutMax=[3]  OutDataTypeStr=uint8  Unit=Cnt
  EPSVoltage : Inport  Port=7  OutMin=[0]  OutMax=[3]  OutDataTypeStr=uint8  Unit=Cnt
  Internal Temp Used : Inport  Port=8  OutMin=[0]  OutMax=[3]  OutDataTypeStr=uint8  Unit=Cnt
  Q-axis Motor Current : Inport  Port=9  OutMin=[0]  OutMax=[3]  OutDataTypeStr=uint8  Unit=Cnt
  Global Real Time from HSCAN : Inport  Port=10  OutMin=[0]  OutMax=[3]  OutDataTypeStr=uint8  Unit=Cnt
  Total Distance from HSCAN : Inport  Port=11  OutMin=[0]  OutMax=[3]  OutDataTypeStr=uint8  Unit=Cnt
  VehSpd : Inport  Port=12  OutMin=[0]  OutMax=[3]  OutDataTypeStr=uint8  Unit=Cnt
  FordVehOutdAirT : Inport  Port=13  OutMin=[0]  OutMax=[3]  OutDataTypeStr=uint8  Unit=Cnt
  FordVehGlbRealTi : Inport  Port=14  OutMin=[0]  OutMax=[3]  OutDataTypeStr=uint8  Unit=Cnt
  Vehicle Data : Inport  Port=15  OutMin=[0]  OutMax=[3]  OutDataTypeStr=uint8  Unit=Cnt
  Ford In House Software Feature Configuration : Inport  Port=16  OutMin=[0]  OutMax=[3]  OutDataTypeStr=uint8  Unit=Cnt
  Feature Configuration : Inport  Port=17  OutMin=[0]  OutMax=[3]  OutDataTypeStr=uint8  Unit=Cnt
  Enable/Disable DTC’s : Inport  Port=18  OutMin=[0]  OutMax=[3]  OutDataTypeStr=uint8  Unit=Cnt
  Developmental Message Configuration : Inport  Port=19  OutMin=[0]  OutMax=[3]  OutDataTypeStr=uint8  Unit=Cnt
  XCP Enable/Disable : Inport  Port=20  OutMin=[0]  OutMax=[3]  OutDataTypeStr=uint8  Unit=Cnt
  Assist on/off : Inport  Port=21  OutMin=[0]  OutMax=[3]  OutDataTypeStr=uint8  Unit=Cnt
  IgnitionCycleCounter : Inport  Port=22  OutMin=[0]  OutMax=[3]  OutDataTypeStr=uint8  Unit=Cnt
  IgnitionOnTime : Inport  Port=23  OutMin=[0]  OutMax=[3]  OutDataTypeStr=uint8  Unit=Cnt
  AppliedFinalMotorTorque : Inport  Port=24  OutMin=[0]  OutMax=[3]  OutDataTypeStr=uint8  Unit=Cnt
  VIN Changed : Inport  Port=25  OutMin=[0]  OutMax=[3]  OutDataTypeStr=uint8  Unit=Cnt
  EPSSystemState : Inport  Port=26  OutMin=[0]  OutMax=[3]  OutDataTypeStr=uint8  Unit=Cnt
  Connected Vehicle: LoA Fault Reporting : Inport  Port=27  OutMin=[0]  OutMax=[3]  OutDataTypeStr=uint8  Unit=Cnt
  Connected Vehicle: Current Level Counters : Inport  Port=28  OutMin=[0]  OutMax=[3]  OutDataTypeStr=uint8  Unit=Cnt
  Connected Vehicle: Voltage Level Counters : Inport  Port=29  OutMin=[0]  OutMax=[3]  OutDataTypeStr=uint8  Unit=Cnt
  Connected Vehicle: Temperature Level Counters : Inport  Port=30  OutMin=[0]  OutMax=[3]  OutDataTypeStr=uint8  Unit=Cnt
  Research Message Configuration : Inport  Port=31  OutMin=[0]  OutMax=[3]  OutDataTypeStr=uint8  Unit=Cnt
  Research Feature Switch : Inport  Port=32  OutMin=[0]  OutMax=[3]  OutDataTypeStr=uint8  Unit=Cnt
  FeaturesActive : Inport  Port=33  OutMin=[0]  OutMax=[3]  OutDataTypeStr=uint8  Unit=Cnt
  SDM_SteeringMode : Inport  Port=34  OutMin=[0]  OutMax=[3]  OutDataTypeStr=uint8  Unit=Cnt
  FIHVersion : Inport  Port=35  OutMin=[0]  OutMax=[3]  OutDataTypeStr=uint8  Unit=Cnt
  ReadSrvActvNiblCmpIntSts : Inport  Port=36
  ReadSrvLaneDprtrWarnIntSts : Inport  Port=37
  ReadSrvLaneKeepAssiIntSts : Inport  Port=38
  ReadSrvLatCtrlIntSts : Inport  Port=39
  ReadSrvPullDriftCmpIntSts : Inport  Port=40
  SrvPullDriftCmpAct : Inport  Port=41
  ReadSrvTrlrBackupAssiIntSts : Inport  Port=42
  ReadSrvFordSteerTqDstbcRejctnIntSts : Inport  Port=43
  ReadSrvFordEvasSteerAssiIntSts : Inport  Port=44
  ReadSrvFordTqSteerCmpActvnCntr : Inport  Port=45
  ReadSrvFordBrkPlsRednActvnCntr : Inport  Port=46
  Supplier Factory Mode : Inport  Port=47  OutMin=[0]  OutMax=[3]  OutDataTypeStr=uint8  Unit=Cnt
  Supplier Internal Fault Code : Inport  Port=48  OutMin=[0]  OutMax=[3]  OutDataTypeStr=uint8  Unit=Cnt
  Supplier Internal Error Memory : Inport  Port=49  OutMin=[0]  OutMax=[3]  OutDataTypeStr=uint8  Unit=Cnt
  ECU Cal-Config Part Number : Inport  Port=50  OutMin=[0]  OutMax=[3]  OutDataTypeStr=uint8  Unit=Cnt
  Subsystem Specific Diagnostic Specification Part Number : Inport  Port=51  OutMin=[0]  OutMax=[3]  OutDataTypeStr=uint8  Unit=Cnt
  ECU Core Assembly Number : Inport  Port=52  OutMin=[0]  OutMax=[3]  OutDataTypeStr=uint8  Unit=Cnt
  ECU Delivery Assembly Number : Inport  Port=53  OutMin=[0]  OutMax=[3]  OutDataTypeStr=uint8  Unit=Cnt
  ECU System Cal-Config Part Number : Inport  Port=54  OutMin=[0]  OutMax=[3]  OutDataTypeStr=uint8  Unit=Cnt
  NOS Generation Tool Version Number : Inport  Port=55  OutMin=[0]  OutMax=[3]  OutDataTypeStr=uint8  Unit=Cnt
  Software Download Specification Version : Inport  Port=56  OutMin=[0]  OutMax=[3]  OutDataTypeStr=uint8  Unit=Cnt
  Diagnostic Specification Version : Inport  Port=57  OutMin=[0]  OutMax=[3]  OutDataTypeStr=uint8  Unit=Cnt
  NOS Message Database #1 Version Number : Inport  Port=58  OutMin=[0]  OutMax=[3]  OutDataTypeStr=uint8  Unit=Cnt
  NOS Boot Loader Generation Tool Version : Inport  Port=59  OutMin=[0]  OutMax=[3]  OutDataTypeStr=uint8  Unit=Cnt
  Boot Software Identification : Inport  Port=60  OutMin=[0]  OutMax=[3]  OutDataTypeStr=uint8  Unit=Cnt
  Vehicle Manufacturer ECU Software Number : Inport  Port=61  OutMin=[0]  OutMax=[3]  OutDataTypeStr=uint8  Unit=Cnt
  System Supplier Identifier : Inport  Port=62  OutMin=[0]  OutMax=[3]  OutDataTypeStr=uint8  Unit=Cnt
  ECU Serial Number : Inport  Port=63  OutMin=[0]  OutMax=[3]  OutDataTypeStr=uint8  Unit=Cnt
  Vehicle Identification Number : Inport  Port=64  OutMin=[0]  OutMax=[3]  OutDataTypeStr=uint8  Unit=Cnt
  WrSrvDrvrSteerRcmdnEnad : Outport
  WrSrvExtAgCtrlEnad : Outport  Port=2
  WrSrvFordAbsPrsnt : Outport  Port=3
  WrSrvFordActvNiblCtrlEnad : Outport  Port=4
  WrSrvFordWrSrvActvParkAssiEnad : Outport  Port=5
  WrSrvFordBrkOscnRednEnad : Outport  Port=6
  WrSrvFordBrkPlsRejctnEnad : Outport  Port=7
  WrSrvFordEvasSteerAssiEnad : Outport  Port=8
  WrSrvFordLaneCentrAssiEnad : Outport  Port=9
  WrSrvFordLaneDprtrWarnEnad : Outport  Port=10
  WrSrvFordLaneKeepAssiEnad : Outport  Port=11
  WrSrvFordPullDriftCmpEnad : Outport  Port=12
  WrSrvFordResrchFctEnad : Outport  Port=13
  WrSrvFordSelctvDrvModEnad : Outport  Port=14
  WrSrvFordTqSteerCmpEnad : Outport  Port=15
  WrSrvFordTrfcJamAssiEnad : Outport  Port=16
  WrSrvFordTrlrBackupAssi5WhlEnad : Outport  Port=17
  WrSrvFordTrlrBackupAssiEnad : Outport  Port=18
  WrSrvFordTrlrBackupAssiTRGEnad : Outport  Port=19
  WrSrvFordVehLoSpdMtnCtrlBrkDecelEna : Outport  Port=20
  WrSrvLaneDetnWarnEnad : Outport  Port=21
  WrSrvActvFrntSteerPrsnt : Outport  Port=22
  WrSrvStrtStopEnadSt : Outport  Port=23
  WrSrvActvRtnEnad : Outport  Port=24
  WrSrvSwEndStopEnad : Outport  Port=25
  WrSrvIgnCycCntr : Outport  Port=26
  WrSrvFordEscPrsnt : Outport  Port=27
  WrSrvLimpHomeDtcCntr : Outport  Port=28
  WrSrvProgsnCntr : Outport  Port=29
  WrSrvHwVrnt : Outport  Port=30
  WrSrvTunVrnt : Outport  Port=31
  WrSrvFordTqSteerCmpActvnCntr : Outport  Port=32
  WrSrvFordBrkPlsRednActvnCntr : Outport  Port=33
  WrSrvSrvPullDriftCmpRstVal : Outport  Port=34
  WrSrvActvNiblCmpIntSts : Outport  Port=35
  WrSrvFordLaneKeepAssiIntSts : Outport  Port=36
  WrSrvPullDriftCmpIntSts : Outport  Port=37
  WrSrvFordLaneDprtrWarnIntSts : Outport  Port=38
  WrSrvFordSteerTqDstbcRejctnIntSts : Outport  Port=39
  WrSrvFordEvasSteerAssiIntSts : Outport  Port=40
  WrSrvLatCtrlIntStsIntSts : Outport  Port=41
  WrSrvTrlrBackupAssiIntSts : Outport  Port=42
  WrSrvFordExtAgCtrlStsInt : Outport  Port=43
  WrSrvEngTqClass : Outport  Port=44
  WrSrvSupplier Factory Mode : Outport  Port=45
  WrSrvResearch Feature Switch : Outport  Port=46
  WrSrvResearch Message Configuration : Outport  Port=47
  WrSrvXCP Enable/Disable : Outport  Port=48
  WrSrvAssist on/off : Outport  Port=49
  WrSrvDevelopmental Message Configuration : Outport  Port=50

== system Ford_T3T6_ArchCnctnDigrm/Ford CFs/Customer Diag Services/CF088A_FordDualEcuFltDiagcCom ==
  EcuId : Inport  OutMin=[0]  OutMax=[3]  OutDataTypeStr=uint8  Unit=Cnt
  Dem_GetEventStatus : Inport  Port=2  OutMin=[0]  OutMax=[1]
  GetSigImcData_u08 : Inport  Port=3  OutMin=[0]  OutMax=[1]
  SetNtcSts : Inport  Port=4  OutMin=[0]  OutMax=[1]
  FordDtcIdx : Outport  OutMin=[0]  OutMax=[255]  OutDataTypeStr=uint8
  FordDtcSts : Outport  Port=2  OutMin=[0]  OutMax=[2558]  OutDataTypeStr=uint8

== system Ford_T3T6_ArchCnctnDigrm/Ford CFs/FIH Read and Write/FIH Initialize ==
  note: ASIL QM FIH
  note: ASIL B FIH
  note: ANC_FunctionCallStatus
      | No Units
      | Bool
      |
      | LKA_FunctionCallStatus
      | No Units
      | Bool
      |
      | LDW_FunctionCallStatus
      | No Units
      | Bool
      |
      | LATCTL_FunctionCallStatus
      | No Units
      | Bool
      |
      | PDC_FunctionCallStatus
      | No Units
      | Bool
      |
      | STDR_FunctionCallStatus
      | No Units
      | Bool
      |
      | ESA_FunctionCallStatus
      | No Units
      | Bool
      |
      | DSR_FunctionCallStatus
      | No Units
      | Bool
  CF061A_FordBlaBoxInitAndFctCall1 : Subsystem  Tag=1.0.X  Description=This function initializes and calls the ASIL QM Ford In House feature functions.
      settings: AttributesFormatString=Version: %<Tag>
  CF093A_FordBlaBoxInitAndFctCall2 : Subsystem  Tag=1.0.X  Description=This function initializes and calls the ASIL B Ford In House feature functions.
      settings: AttributesFormatString=Version: %<Tag>
  tag scope: ActvNiblCtrlFctCallSts=global, EvasSteerAssiFctCallSts=global, FordLaneKeepAssiFctCallSts=global, LaneDprtrWarnFctCallSts=global, LatCtrlFctCallSts=global, PullDriftCmpFctCallSts=global, SteerTqDstbcRejctnFctCallSts=global
  wires:
  [EcuId] -> CF093A_FordBlaBoxInitAndFctCall2/1(EcuId)
  [FordEpsSysSt] -> CF093A_FordBlaBoxInitAndFctCall2/2(FordEpsSysSt)
  [FordEvasSteerAssiEnad] -> CF093A_FordBlaBoxInitAndFctCall2/3(FordEvasSteerAssiEna)
  [SteerTqDstbcRejctnEna] -> CF093A_FordBlaBoxInitAndFctCall2/4(SteerTqDstbcRejctnEna)
  CF093A_FordBlaBoxInitAndFctCall2/1(EvasSteerAssiFctCallSts) -> [EvasSteerAssiFctCallSts]
  CF093A_FordBlaBoxInitAndFctCall2/2(SteerTqDstbcRejctnFctCallSts) -> [SteerTqDstbcRejctnFctCallSts]
  [EcuId] -> CF061A_FordBlaBoxInitAndFctCall1/1(EcuId)
  [FordActvNiblCtrlEnad] -> CF061A_FordBlaBoxInitAndFctCall1/2(FordActvNiblCtrlEnad)
  [FordEpsSysSt] -> CF061A_FordBlaBoxInitAndFctCall1/3(FordEpsSysSt)
  [FordLaneDprtrWarnEnad] -> CF061A_FordBlaBoxInitAndFctCall1/4(FordLaneDprtrWarnEnad)
  [FordLaneKeepAssiEnad] -> CF061A_FordBlaBoxInitAndFctCall1/5(FordLaneKeepingAssiEnad)
  [FordPullDriftCmpEnad] -> CF061A_FordBlaBoxInitAndFctCall1/6(FordPullDriftCmpEnad)
  [FordTrlrBackupAssiEnad] -> CF061A_FordBlaBoxInitAndFctCall1/7(FordTrlrBackupAssiEnad)
  CF061A_FordBlaBoxInitAndFctCall1/1(ActvNiblCtrlFctCallSts) -> [ActvNiblCtrlFctCallSts]
  CF061A_FordBlaBoxInitAndFctCall1/2(FordLaneKeepingAssiFctCallSts) -> [FordLaneKeepAssiFctCallSts]
  CF061A_FordBlaBoxInitAndFctCall1/3(LaneDprtrWarnFctCallSts) -> [LaneDprtrWarnFctCallSts]
  CF061A_FordBlaBoxInitAndFctCall1/4(LatCtrlFctCallSts) -> [LatCtrlFctCallSts]
  CF061A_FordBlaBoxInitAndFctCall1/5(PullDriftCmpFctCallSts) -> [PullDriftCmpFctCallSts]
